simulink model "carry_ripple_adder"  (R2022b)
settings: Solver=FixedStepDiscrete  StartTime=0.0  StopTime=10  RelTol=1e-3
PreLoadFcn:
  | addpath('C:\Course_Material\UofT\ECE1718\assignment2\matlab_tests\hdlimport\carry_ripple_adder');
libraries: simulink x188, hdlsllib x65
(part 1 of 2)
CloseFcn:
  | addpath('C:\Course_Material\UofT\ECE1718\assignment2\matlab_tests\hdlimport\carry_ripple_adder');
  | rmpath('C:\Course_Material\UofT\ECE1718\assignment2\matlab_tests\hdlimport\carry_ripple_adder');
settings Model: DataTypeOverride=Off  Creator=13698  LastModifiedBy=13698
settings OptimizationCC: BlockReduction=off  ConditionallyExecuteInputs=off  DefaultParameterBehavior=Inlined  InheritOutputTypeSmallerThanSingle=on
settings DebuggingCC: AlgebraicLoopMsg=error  InheritedTsInSrcMsg=none  SingleTaskRateTransMsg=error
settings HardwareCC: ProdBitPerPointer=32  ProdBitPerSizeT=32  ProdBitPerPtrDiffT=32  ProdLargestAtomicFloat=None  ProdIntDivRoundTo=Undefined  ProdEndianess=Unspecified  ProdWordSize=32  ProdHWDeviceType=ASIC/FPGA->ASIC/FPGA  TargetBitPerPointer=64  TargetBitPerSizeT=64  TargetBitPerPtrDiffT=64  TargetLongLongMode=on  TargetIntDivRoundTo=Zero  TargetEndianess=LittleEndian  TargetWordSize=64  TargetHWDeviceType=Custom Processor->MATLAB Host Computer  ProdEqTarget=off

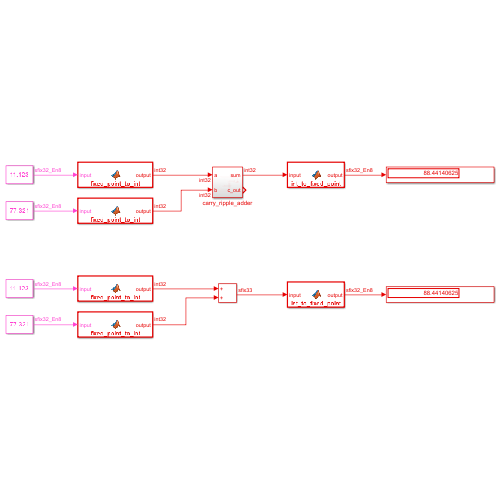
[thumbnail: Simulink's stored preview of the top-level diagram]
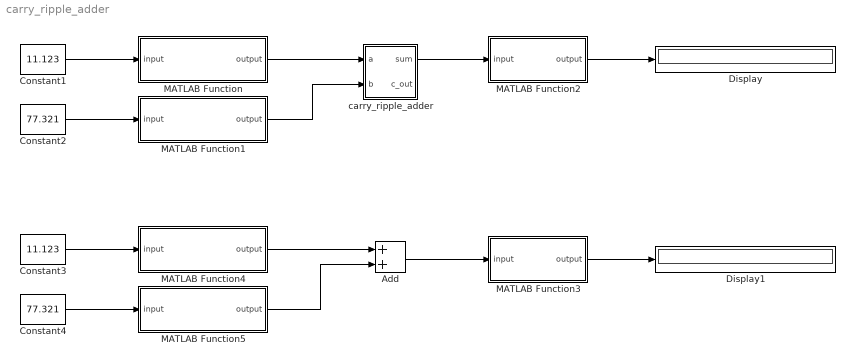
== system carry_ripple_adder ==
  Add : Sum
  Constant1 : Constant  Value=11.123  OutDataTypeStr=fixdt(1,32,8)
  Constant2 : Constant  Value=77.321  OutDataTypeStr=fixdt(1,32,8)
  Constant3 : Constant  Value=11.123  OutDataTypeStr=fixdt(1,32,8)
  Constant4 : Constant  Value=77.321  OutDataTypeStr=fixdt(1,32,8)
  Display : Display
  Display1 : Display
  MATLAB Function : MATLAB Function  TreatAsAtomicUnit=on
  MATLAB Function1 : MATLAB Function  TreatAsAtomicUnit=on
  MATLAB Function2 : MATLAB Function  TreatAsAtomicUnit=on
  MATLAB Function3 : MATLAB Function  TreatAsAtomicUnit=on
  MATLAB Function4 : MATLAB Function  TreatAsAtomicUnit=on
  MATLAB Function5 : MATLAB Function  TreatAsAtomicUnit=on
  carry_ripple_adder : Subsystem
  wires:
  MATLAB Function/1(output) -> carry_ripple_adder/1(a)
  MATLAB Function1/1(output) -> carry_ripple_adder/2(b)
  carry_ripple_adder/1(sum) -> MATLAB Function2/1(input)
  Constant1/1 -> MATLAB Function/1(input)
  MATLAB Function2/1(output) -> Display/1
  Add/1 -> MATLAB Function3/1(input)
  MATLAB Function3/1(output) -> Display1/1
  Constant3/1 -> MATLAB Function4/1(input)
  MATLAB Function4/1(output) -> Add/1
  MATLAB Function5/1(output) -> Add/2
  Constant2/1 -> MATLAB Function1/1(input)
  Constant4/1 -> MATLAB Function5/1(input)

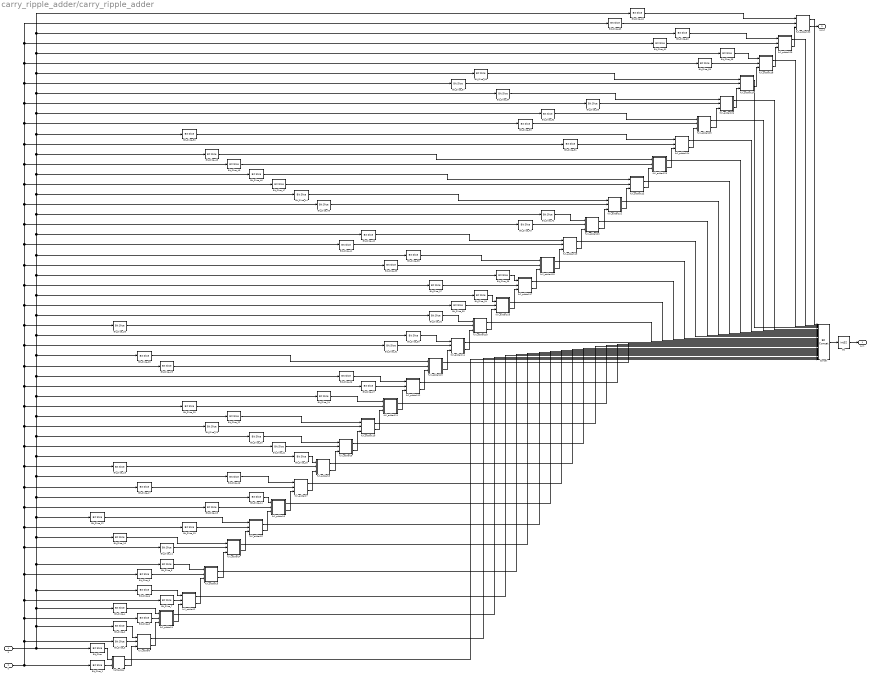
== system carry_ripple_adder/carry_ripple_adder ==
  a : Inport  OutDataTypeStr=int32  SampleTime=-1
  b : Inport  Port=2  OutDataTypeStr=int32  SampleTime=-1
  Bit_Slice : hdlsllib/Logic and Bit Operations/Bit Slice  lidx=double(0)  ridx=double(0)
  Bit_Slice_1 : hdlsllib/Logic and Bit Operations/Bit Slice  lidx=double(0)  ridx=double(0)
  Bit_Slice_10 : hdlsllib/Logic and Bit Operations/Bit Slice  lidx=double(5)  ridx=double(5)
  Bit_Slice_11 : hdlsllib/Logic and Bit Operations/Bit Slice  lidx=double(5)  ridx=double(5)
  Bit_Slice_12 : hdlsllib/Logic and Bit Operations/Bit Slice  lidx=double(6)  ridx=double(6)
  Bit_Slice_13 : hdlsllib/Logic and Bit Operations/Bit Slice  lidx=double(6)  ridx=double(6)
  Bit_Slice_14 : hdlsllib/Logic and Bit Operations/Bit Slice  lidx=double(7)  ridx=double(7)
  Bit_Slice_15 : hdlsllib/Logic and Bit Operations/Bit Slice  lidx=double(7)  ridx=double(7)
  Bit_Slice_16 : hdlsllib/Logic and Bit Operations/Bit Slice  lidx=double(8)  ridx=double(8)
  Bit_Slice_17 : hdlsllib/Logic and Bit Operations/Bit Slice  lidx=double(8)  ridx=double(8)
  Bit_Slice_18 : hdlsllib/Logic and Bit Operations/Bit Slice  lidx=double(9)  ridx=double(9)
  Bit_Slice_19 : hdlsllib/Logic and Bit Operations/Bit Slice  lidx=double(9)  ridx=double(9)
  Bit_Slice_2 : hdlsllib/Logic and Bit Operations/Bit Slice  lidx=double(1)  ridx=double(1)
  Bit_Slice_20 : hdlsllib/Logic and Bit Operations/Bit Slice  lidx=double(10)  ridx=double(10)
  Bit_Slice_21 : hdlsllib/Logic and Bit Operations/Bit Slice  lidx=double(10)  ridx=double(10)
  Bit_Slice_22 : hdlsllib/Logic and Bit Operations/Bit Slice  lidx=double(11)  ridx=double(11)
  Bit_Slice_23 : hdlsllib/Logic and Bit Operations/Bit Slice  lidx=double(11)  ridx=double(11)
  Bit_Slice_24 : hdlsllib/Logic and Bit Operations/Bit Slice  lidx=double(12)  ridx=double(12)
  Bit_Slice_25 : hdlsllib/Logic and Bit Operations/Bit Slice  lidx=double(12)  ridx=double(12)
  Bit_Slice_26 : hdlsllib/Logic and Bit Operations/Bit Slice  lidx=double(13)  ridx=double(13)
  Bit_Slice_27 : hdlsllib/Logic and Bit Operations/Bit Slice  lidx=double(13)  ridx=double(13)
  Bit_Slice_28 : hdlsllib/Logic and Bit Operations/Bit Slice  lidx=double(14)  ridx=double(14)
  Bit_Slice_29 : hdlsllib/Logic and Bit Operations/Bit Slice  lidx=double(14)  ridx=double(14)
  Bit_Slice_3 : hdlsllib/Logic and Bit Operations/Bit Slice  lidx=double(1)  ridx=double(1)
  Bit_Slice_30 : hdlsllib/Logic and Bit Operations/Bit Slice  lidx=double(15)  ridx=double(15)
  Bit_Slice_31 : hdlsllib/Logic and Bit Operations/Bit Slice  lidx=double(15)  ridx=double(15)
  Bit_Slice_32 : hdlsllib/Logic and Bit Operations/Bit Slice  lidx=double(16)  ridx=double(16)
  Bit_Slice_33 : hdlsllib/Logic and Bit Operations/Bit Slice  lidx=double(16)  ridx=double(16)
  Bit_Slice_34 : hdlsllib/Logic and Bit Operations/Bit Slice  lidx=double(17)  ridx=double(17)
  Bit_Slice_35 : hdlsllib/Logic and Bit Operations/Bit Slice  lidx=double(17)  ridx=double(17)
  Bit_Slice_36 : hdlsllib/Logic and Bit Operations/Bit Slice  lidx=double(18)  ridx=double(18)
  Bit_Slice_37 : hdlsllib/Logic and Bit Operations/Bit Slice  lidx=double(18)  ridx=double(18)
  Bit_Slice_38 : hdlsllib/Logic and Bit Operations/Bit Slice  lidx=double(19)  ridx=double(19)
  Bit_Slice_39 : hdlsllib/Logic and Bit Operations/Bit Slice  lidx=double(19)  ridx=double(19)
  Bit_Slice_4 : hdlsllib/Logic and Bit Operations/Bit Slice  lidx=double(2)  ridx=double(2)
  Bit_Slice_40 : hdlsllib/Logic and Bit Operations/Bit Slice  lidx=double(20)  ridx=double(20)
  Bit_Slice_41 : hdlsllib/Logic and Bit Operations/Bit Slice  lidx=double(20)  ridx=double(20)
  Bit_Slice_42 : hdlsllib/Logic and Bit Operations/Bit Slice  lidx=double(21)  ridx=double(21)
  Bit_Slice_43 : hdlsllib/Logic and Bit Operations/Bit Slice  lidx=double(21)  ridx=double(21)
  Bit_Slice_44 : hdlsllib/Logic and Bit Operations/Bit Slice  lidx=double(22)  ridx=double(22)
  Bit_Slice_45 : hdlsllib/Logic and Bit Operations/Bit Slice  lidx=double(22)  ridx=double(22)
  Bit_Slice_46 : hdlsllib/Logic and Bit Operations/Bit Slice  lidx=double(23)  ridx=double(23)
  Bit_Slice_47 : hdlsllib/Logic and Bit Operations/Bit Slice  lidx=double(23)  ridx=double(23)
  Bit_Slice_48 : hdlsllib/Logic and Bit Operations/Bit Slice  lidx=double(24)  ridx=double(24)
  Bit_Slice_49 : hdlsllib/Logic and Bit Operations/Bit Slice  lidx=double(24)  ridx=double(24)
  Bit_Slice_5 : hdlsllib/Logic and Bit Operations/Bit Slice  lidx=double(2)  ridx=double(2)
  Bit_Slice_50 : hdlsllib/Logic and Bit Operations/Bit Slice  lidx=double(25)  ridx=double(25)
  Bit_Slice_51 : hdlsllib/Logic and Bit Operations/Bit Slice  lidx=double(25)  ridx=double(25)
  Bit_Slice_52 : hdlsllib/Logic and Bit Operations/Bit Slice  lidx=double(26)  ridx=double(26)
  Bit_Slice_53 : hdlsllib/Logic and Bit Operations/Bit Slice  lidx=double(26)  ridx=double(26)
  Bit_Slice_54 : hdlsllib/Logic and Bit Operations/Bit Slice  lidx=double(27)  ridx=double(27)
  Bit_Slice_55 : hdlsllib/Logic and Bit Operations/Bit Slice  lidx=double(27)  ridx=double(27)
  Bit_Slice_56 : hdlsllib/Logic and Bit Operations/Bit Slice  lidx=double(28)  ridx=double(28)
  Bit_Slice_57 : hdlsllib/Logic and Bit Operations/Bit Slice  lidx=double(28)  ridx=double(28)
  Bit_Slice_58 : hdlsllib/Logic and Bit Operations/Bit Slice  lidx=double(29)  ridx=double(29)
  Bit_Slice_59 : hdlsllib/Logic and Bit Operations/Bit Slice  lidx=double(29)  ridx=double(29)
  Bit_Slice_6 : hdlsllib/Logic and Bit Operations/Bit Slice  lidx=double(3)  ridx=double(3)
  Bit_Slice_60 : hdlsllib/Logic and Bit Operations/Bit Slice  lidx=double(30)  ridx=double(30)
  Bit_Slice_61 : hdlsllib/Logic and Bit Operations/Bit Slice  lidx=double(30)  ridx=double(30)
  Bit_Slice_62 : hdlsllib/Logic and Bit Operations/Bit Slice  lidx=double(31)  ridx=double(31)
  Bit_Slice_63 : hdlsllib/Logic and Bit Operations/Bit Slice  lidx=double(31)  ridx=double(31)
  Bit_Slice_7 : hdlsllib/Logic and Bit Operations/Bit Slice  lidx=double(3)  ridx=double(3)
  Bit_Slice_8 : hdlsllib/Logic and Bit Operations/Bit Slice  lidx=double(4)  ridx=double(4)
  Bit_Slice_9 : hdlsllib/Logic and Bit Operations/Bit Slice  lidx=double(4)  ridx=double(4)
  Concat : hdlsllib/Logic and Bit Operations/Bit Concat  numInputs=32
  dtc : DataTypeConversion  OutDataTypeStr=int32  ConvertRealWorld=Stored Integer (SI)  SampleTime=-1  SaturateOnIntegerOverflow=off  RndMeth=Floor
  full_adder0 : Subsystem
  full_adder11 : Subsystem
  full_adder110 : Subsystem
  full_adder111 : Subsystem
  full_adder112 : Subsystem
  full_adder113 : Subsystem
  full_adder114 : Subsystem
  full_adder115 : Subsystem
  full_adder116 : Subsystem
  full_adder117 : Subsystem
  full_adder118 : Subsystem
  full_adder119 : Subsystem
  full_adder12 : Subsystem
  full_adder120 : Subsystem
  full_adder121 : Subsystem
  full_adder122 : Subsystem
  full_adder123 : Subsystem
  full_adder124 : Subsystem
  full_adder125 : Subsystem
  full_adder126 : Subsystem
  full_adder127 : Subsystem
  full_adder128 : Subsystem
  full_adder129 : Subsystem
  full_adder13 : Subsystem
  full_adder130 : Subsystem
  full_adder14 : Subsystem
  full_adder15 : Subsystem
  full_adder16 : Subsystem
  full_adder17 : Subsystem
  full_adder18 : Subsystem
  full_adder19 : Subsystem
  half_adder : Subsystem
  sum : Outport  OutDataTypeStr=int32  SampleTime=-1
  c_out : Outport  Port=2  OutDataTypeStr=fixdt(0, 1, 0)  SampleTime=-1
  wires:
  Bit_Slice/1 -> half_adder/1(a)
  full_adder122/2(c_out) -> full_adder123/3(c_in)
  full_adder130/2(c_out) -> c_out/1
  full_adder118/1(sum) -> Concat/13
  full_adder130/1(sum) -> Concat/1
  Bit_Slice_7/1 -> full_adder12/2(b)
  full_adder129/2(c_out) -> full_adder130/3(c_in)
  full_adder0/1(sum) -> Concat/31
  full_adder124/2(c_out) -> full_adder125/3(c_in)
  Concat/1 -> dtc/1
  Bit_Slice_20/1 -> full_adder19/1(a)
  full_adder14/2(c_out) -> full_adder15/3(c_in)
  full_adder117/2(c_out) -> full_adder118/3(c_in)
  full_adder121/2(c_out) -> full_adder122/3(c_in)
  full_adder120/1(sum) -> Concat/11
  full_adder116/1(sum) -> Concat/15
  Bit_Slice_51/1 -> full_adder124/2(b)
  full_adder128/2(c_out) -> full_adder129/3(c_in)
  Bit_Slice_36/1 -> full_adder117/1(a)
  Bit_Slice_28/1 -> full_adder113/1(a)
  Bit_Slice_16/1 -> full_adder17/1(a)
  full_adder120/2(c_out) -> full_adder121/3(c_in)
  full_adder125/2(c_out) -> full_adder126/3(c_in)
  full_adder118/2(c_out) -> full_adder119/3(c_in)
  full_adder12/1(sum) -> Concat/29
  Bit_Slice_18/1 -> full_adder18/1(a)
  full_adder127/2(c_out) -> full_adder128/3(c_in)
  full_adder19/2(c_out) -> full_adder110/3(c_in)
  full_adder126/2(c_out) -> full_adder127/3(c_in)
  full_adder12/2(c_out) -> full_adder13/3(c_in)
  Bit_Slice_14/1 -> full_adder16/1(a)
  full_adder110/2(c_out) -> full_adder111/3(c_in)
  b/1 -> Bit_Slice_63/1, Bit_Slice_61/1, Bit_Slice_59/1, Bit_Slice_57/1, Bit_Slice_55/1, Bit_Slice_53/1, Bit_Slice_51/1, Bit_Slice_49/1, Bit_Slice_47/1, Bit_Slice_45/1, Bit_Slice_43/1, Bit_Slice_41/1, Bit_Slice_39/1, Bit_Slice_37/1, Bit_Slice_35/1, Bit_Slice_33/1, Bit_Slice_31/1, Bit_Slice_29/1, Bit_Slice_27/1, Bit_Slice_25/1, Bit_Slice_23/1, Bit_Slice_21/1, Bit_Slice_19/1, Bit_Slice_17/1, Bit_Slice_15/1, Bit_Slice_13/1, Bit_Slice_11/1, Bit_Slice_9/1, Bit_Slice_7/1, Bit_Slice_5/1, Bit_Slice_3/1, Bit_Slice_1/1
  full_adder119/1(sum) -> Concat/12
  Bit_Slice_34/1 -> full_adder116/1(a)
  full_adder123/2(c_out) -> full_adder124/3(c_in)
  full_adder119/2(c_out) -> full_adder120/3(c_in)
  full_adder0/2(c_out) -> full_adder11/3(c_in)
  a/1 -> Bit_Slice_62/1, Bit_Slice_60/1, Bit_Slice_58/1, Bit_Slice_56/1, Bit_Slice_54/1, Bit_Slice_52/1, Bit_Slice_50/1, Bit_Slice_48/1, Bit_Slice_46/1, Bit_Slice_44/1, Bit_Slice_42/1, Bit_Slice_40/1, Bit_Slice_38/1, Bit_Slice_36/1, Bit_Slice_34/1, Bit_Slice_32/1, Bit_Slice_30/1, Bit_Slice_28/1, Bit_Slice_26/1, Bit_Slice_24/1, Bit_Slice_22/1, Bit_Slice_20/1, Bit_Slice_18/1, Bit_Slice_16/1, Bit_Slice_14/1, Bit_Slice_12/1, Bit_Slice_10/1, Bit_Slice_8/1, Bit_Slice_6/1, Bit_Slice_4/1, Bit_Slice_2/1, Bit_Slice/1
  full_adder116/2(c_out) -> full_adder117/3(c_in)
  Bit_Slice_46/1 -> full_adder122/1(a)
  Bit_Slice_2/1 -> full_adder0/1(a)
  full_adder115/2(c_out) -> full_adder116/3(c_in)
  Bit_Slice_33/1 -> full_adder115/2(b)
  full_adder112/2(c_out) -> full_adder113/3(c_in)
  Bit_Slice_13/1 -> full_adder15/2(b)
  full_adder114/2(c_out) -> full_adder115/3(c_in)
  full_adder113/2(c_out) -> full_adder114/3(c_in)
  full_adder111/2(c_out) -> full_adder112/3(c_in)
  full_adder18/2(c_out) -> full_adder19/3(c_in)
  full_adder123/1(sum) -> Concat/8
  full_adder17/2(c_out) -> full_adder18/3(c_in)
  full_adder13/2(c_out) -> full_adder14/3(c_in)
  Bit_Slice_9/1 -> full_adder13/2(b)
  full_adder16/2(c_out) -> full_adder17/3(c_in)
  full_adder15/2(c_out) -> full_adder16/3(c_in)
  Bit_Slice_3/1 -> full_adder0/2(b)
  full_adder11/2(c_out) -> full_adder12/3(c_in)
  Bit_Slice_5/1 -> full_adder11/2(b)
  Bit_Slice_1/1 -> half_adder/2(b)
  full_adder129/1(sum) -> Concat/2
  half_adder/2(c_out) -> full_adder0/3(c_in)
  full_adder17/1(sum) -> Concat/24
  dtc/1 -> sum/1
  full_adder113/1(sum) -> Concat/18
  Bit_Slice_31/1 -> full_adder114/2(b)
  full_adder124/1(sum) -> Concat/7
  Bit_Slice_10/1 -> full_adder14/1(a)
  Bit_Slice_12/1 -> full_adder15/1(a)
  Bit_Slice_17/1 -> full_adder17/2(b)
  Bit_Slice_19/1 -> full_adder18/2(b)
  Bit_Slice_4/1 -> full_adder11/1(a)
  half_adder/1(sum) -> Concat/32
  Bit_Slice_6/1 -> full_adder12/1(a)
  Bit_Slice_11/1 -> full_adder14/2(b)
  Bit_Slice_29/1 -> full_adder113/2(b)
  Bit_Slice_8/1 -> full_adder13/1(a)
  full_adder125/1(sum) -> Concat/6
  full_adder111/1(sum) -> Concat/20
  full_adder11/1(sum) -> Concat/30
  Bit_Slice_25/1 -> full_adder111/2(b)
  Bit_Slice_50/1 -> full_adder124/1(a)
  Bit_Slice_15/1 -> full_adder16/2(b)
  Bit_Slice_23/1 -> full_adder110/2(b)
  full_adder114/1(sum) -> Concat/17
  Bit_Slice_48/1 -> full_adder123/1(a)
  full_adder13/1(sum) -> Concat/28
  Bit_Slice_22/1 -> full_adder110/1(a)
  Bit_Slice_49/1 -> full_adder123/2(b)
  full_adder14/1(sum) -> Concat/27
  full_adder15/1(sum) -> Concat/26
  Bit_Slice_21/1 -> full_adder19/2(b)
  Bit_Slice_47/1 -> full_adder122/2(b)
  full_adder16/1(sum) -> Concat/25
  Bit_Slice_44/1 -> full_adder121/1(a)
  Bit_Slice_24/1 -> full_adder111/1(a)
  Bit_Slice_45/1 -> full_adder121/2(b)
  full_adder18/1(sum) -> Concat/23
  Bit_Slice_26/1 -> full_adder112/1(a)
  Bit_Slice_41/1 -> full_adder119/2(b)
  full_adder110/1(sum) -> Concat/21
  full_adder19/1(sum) -> Concat/22
  Bit_Slice_27/1 -> full_adder112/2(b)
  Bit_Slice_40/1 -> full_adder119/1(a)
  Bit_Slice_61/1 -> full_adder129/2(b)
  Bit_Slice_39/1 -> full_adder118/2(b)
  Bit_Slice_30/1 -> full_adder114/1(a)
  Bit_Slice_38/1 -> full_adder118/1(a)
  full_adder112/1(sum) -> Concat/19
  Bit_Slice_63/1 -> full_adder130/2(b)
  Bit_Slice_32/1 -> full_adder115/1(a)
  Bit_Slice_37/1 -> full_adder117/2(b)
  Bit_Slice_35/1 -> full_adder116/2(b)
  Bit_Slice_57/1 -> full_adder127/2(b)
  Bit_Slice_56/1 -> full_adder127/1(a)
  Bit_Slice_58/1 -> full_adder128/1(a)
  full_adder115/1(sum) -> Concat/16
  Bit_Slice_54/1 -> full_adder126/1(a)
  Bit_Slice_43/1 -> full_adder120/2(b)
  Bit_Slice_53/1 -> full_adder125/2(b)
  full_adder117/1(sum) -> Concat/14
  Bit_Slice_42/1 -> full_adder120/1(a)
  Bit_Slice_52/1 -> full_adder125/1(a)
  Bit_Slice_60/1 -> full_adder129/1(a)
  Bit_Slice_55/1 -> full_adder126/2(b)
  full_adder121/1(sum) -> Concat/10
  Bit_Slice_62/1 -> full_adder130/1(a)
  full_adder122/1(sum) -> Concat/9
  Bit_Slice_59/1 -> full_adder128/2(b)
  full_adder126/1(sum) -> Concat/5
  full_adder127/1(sum) -> Concat/4
  full_adder128/1(sum) -> Concat/3

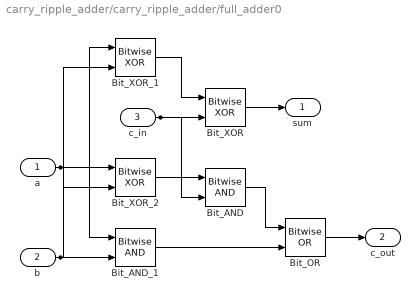
== system carry_ripple_adder/carry_ripple_adder/full_adder0 ==
  a : Inport  OutDataTypeStr=fixdt(0, 1, 0)  SampleTime=-1
  b : Inport  Port=2  OutDataTypeStr=fixdt(0, 1, 0)  SampleTime=-1
  c_in : Inport  Port=3  OutDataTypeStr=fixdt(0, 1, 0)  SampleTime=-1
  Bit_AND : simulink/Logic and Bit Operations/Bitwise Operator  logicop=AND  UseBitMask=off  NumInputPorts=2  BitMask=double(0)  BitMaskRealWorld=Real World Value
  Bit_AND_1 : simulink/Logic and Bit Operations/Bitwise Operator  logicop=AND  UseBitMask=off  NumInputPorts=2  BitMask=double(0)  BitMaskRealWorld=Real World Value
  Bit_OR : simulink/Logic and Bit Operations/Bitwise Operator  logicop=OR  UseBitMask=off  NumInputPorts=2  BitMask=double(0)  BitMaskRealWorld=Real World Value
  Bit_XOR : simulink/Logic and Bit Operations/Bitwise Operator  logicop=XOR  UseBitMask=off  NumInputPorts=2  BitMask=double(0)  BitMaskRealWorld=Real World Value
  Bit_XOR_1 : simulink/Logic and Bit Operations/Bitwise Operator  logicop=XOR  UseBitMask=off  NumInputPorts=2  BitMask=double(0)  BitMaskRealWorld=Real World Value
  Bit_XOR_2 : simulink/Logic and Bit Operations/Bitwise Operator  logicop=XOR  UseBitMask=off  NumInputPorts=2  BitMask=double(0)  BitMaskRealWorld=Real World Value
  sum : Outport  OutDataTypeStr=fixdt(0, 1, 0)  SampleTime=-1
  c_out : Outport  Port=2  OutDataTypeStr=fixdt(0, 1, 0)  SampleTime=-1
  wires:
  a/1 -> Bit_XOR_2/1, Bit_XOR_1/1, Bit_AND_1/1
  b/1 -> Bit_AND_1/2, Bit_XOR_2/2, Bit_XOR_1/2
  Bit_AND/1 -> Bit_OR/1
  Bit_XOR/1 -> sum/1
  Bit_AND_1/1 -> Bit_OR/2
  Bit_XOR_2/1 -> Bit_AND/1
  Bit_XOR_1/1 -> Bit_XOR/1
  c_in/1 -> Bit_AND/2, Bit_XOR/2
  Bit_OR/1 -> c_out/1

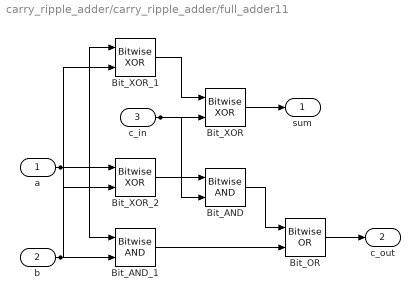
== system carry_ripple_adder/carry_ripple_adder/full_adder11 ==
  a : Inport  OutDataTypeStr=fixdt(0, 1, 0)  SampleTime=-1
  b : Inport  Port=2  OutDataTypeStr=fixdt(0, 1, 0)  SampleTime=-1
  c_in : Inport  Port=3  OutDataTypeStr=fixdt(0, 1, 0)  SampleTime=-1
  Bit_AND : simulink/Logic and Bit Operations/Bitwise Operator  logicop=AND  UseBitMask=off  NumInputPorts=2  BitMask=double(0)  BitMaskRealWorld=Real World Value
  Bit_AND_1 : simulink/Logic and Bit Operations/Bitwise Operator  logicop=AND  UseBitMask=off  NumInputPorts=2  BitMask=double(0)  BitMaskRealWorld=Real World Value
  Bit_OR : simulink/Logic and Bit Operations/Bitwise Operator  logicop=OR  UseBitMask=off  NumInputPorts=2  BitMask=double(0)  BitMaskRealWorld=Real World Value
  Bit_XOR : simulink/Logic and Bit Operations/Bitwise Operator  logicop=XOR  UseBitMask=off  NumInputPorts=2  BitMask=double(0)  BitMaskRealWorld=Real World Value
  Bit_XOR_1 : simulink/Logic and Bit Operations/Bitwise Operator  logicop=XOR  UseBitMask=off  NumInputPorts=2  BitMask=double(0)  BitMaskRealWorld=Real World Value
  Bit_XOR_2 : simulink/Logic and Bit Operations/Bitwise Operator  logicop=XOR  UseBitMask=off  NumInputPorts=2  BitMask=double(0)  BitMaskRealWorld=Real World Value
  sum : Outport  OutDataTypeStr=fixdt(0, 1, 0)  SampleTime=-1
  c_out : Outport  Port=2  OutDataTypeStr=fixdt(0, 1, 0)  SampleTime=-1
  wires:
  a/1 -> Bit_XOR_2/1, Bit_XOR_1/1, Bit_AND_1/1
  b/1 -> Bit_AND_1/2, Bit_XOR_2/2, Bit_XOR_1/2
  Bit_AND/1 -> Bit_OR/1
  Bit_XOR/1 -> sum/1
  Bit_AND_1/1 -> Bit_OR/2
  Bit_XOR_2/1 -> Bit_AND/1
  Bit_XOR_1/1 -> Bit_XOR/1
  c_in/1 -> Bit_AND/2, Bit_XOR/2
  Bit_OR/1 -> c_out/1

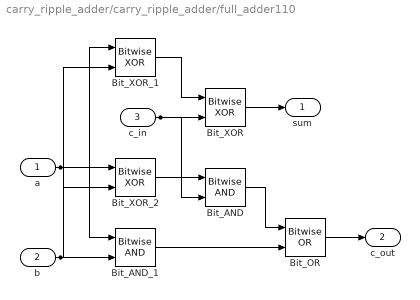
== system carry_ripple_adder/carry_ripple_adder/full_adder110 ==
  a : Inport  OutDataTypeStr=fixdt(0, 1, 0)  SampleTime=-1
  b : Inport  Port=2  OutDataTypeStr=fixdt(0, 1, 0)  SampleTime=-1
  c_in : Inport  Port=3  OutDataTypeStr=fixdt(0, 1, 0)  SampleTime=-1
  Bit_AND : simulink/Logic and Bit Operations/Bitwise Operator  logicop=AND  UseBitMask=off  NumInputPorts=2  BitMask=double(0)  BitMaskRealWorld=Real World Value
  Bit_AND_1 : simulink/Logic and Bit Operations/Bitwise Operator  logicop=AND  UseBitMask=off  NumInputPorts=2  BitMask=double(0)  BitMaskRealWorld=Real World Value
  Bit_OR : simulink/Logic and Bit Operations/Bitwise Operator  logicop=OR  UseBitMask=off  NumInputPorts=2  BitMask=double(0)  BitMaskRealWorld=Real World Value
  Bit_XOR : simulink/Logic and Bit Operations/Bitwise Operator  logicop=XOR  UseBitMask=off  NumInputPorts=2  BitMask=double(0)  BitMaskRealWorld=Real World Value
  Bit_XOR_1 : simulink/Logic and Bit Operations/Bitwise Operator  logicop=XOR  UseBitMask=off  NumInputPorts=2  BitMask=double(0)  BitMaskRealWorld=Real World Value
  Bit_XOR_2 : simulink/Logic and Bit Operations/Bitwise Operator  logicop=XOR  UseBitMask=off  NumInputPorts=2  BitMask=double(0)  BitMaskRealWorld=Real World Value
  sum : Outport  OutDataTypeStr=fixdt(0, 1, 0)  SampleTime=-1
  c_out : Outport  Port=2  OutDataTypeStr=fixdt(0, 1, 0)  SampleTime=-1
  wires:
  Bit_AND/1 -> Bit_OR/1
  Bit_XOR/1 -> sum/1
  Bit_AND_1/1 -> Bit_OR/2
  a/1 -> Bit_AND_1/1, Bit_XOR_2/1, Bit_XOR_1/1
  Bit_XOR_2/1 -> Bit_AND/1
  Bit_XOR_1/1 -> Bit_XOR/1
  b/1 -> Bit_AND_1/2, Bit_XOR_2/2, Bit_XOR_1/2
  c_in/1 -> Bit_AND/2, Bit_XOR/2
  Bit_OR/1 -> c_out/1

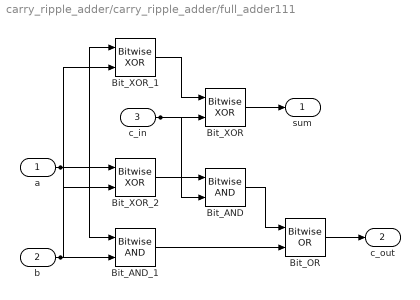
== system carry_ripple_adder/carry_ripple_adder/full_adder111 ==
  a : Inport  OutDataTypeStr=fixdt(0, 1, 0)  SampleTime=-1
  b : Inport  Port=2  OutDataTypeStr=fixdt(0, 1, 0)  SampleTime=-1
  c_in : Inport  Port=3  OutDataTypeStr=fixdt(0, 1, 0)  SampleTime=-1
  Bit_AND : simulink/Logic and Bit Operations/Bitwise Operator  logicop=AND  UseBitMask=off  NumInputPorts=2  BitMask=double(0)  BitMaskRealWorld=Real World Value
  Bit_AND_1 : simulink/Logic and Bit Operations/Bitwise Operator  logicop=AND  UseBitMask=off  NumInputPorts=2  BitMask=double(0)  BitMaskRealWorld=Real World Value
  Bit_OR : simulink/Logic and Bit Operations/Bitwise Operator  logicop=OR  UseBitMask=off  NumInputPorts=2  BitMask=double(0)  BitMaskRealWorld=Real World Value
  Bit_XOR : simulink/Logic and Bit Operations/Bitwise Operator  logicop=XOR  UseBitMask=off  NumInputPorts=2  BitMask=double(0)  BitMaskRealWorld=Real World Value
  Bit_XOR_1 : simulink/Logic and Bit Operations/Bitwise Operator  logicop=XOR  UseBitMask=off  NumInputPorts=2  BitMask=double(0)  BitMaskRealWorld=Real World Value
  Bit_XOR_2 : simulink/Logic and Bit Operations/Bitwise Operator  logicop=XOR  UseBitMask=off  NumInputPorts=2  BitMask=double(0)  BitMaskRealWorld=Real World Value
  sum : Outport  OutDataTypeStr=fixdt(0, 1, 0)  SampleTime=-1
  c_out : Outport  Port=2  OutDataTypeStr=fixdt(0, 1, 0)  SampleTime=-1
  wires:
  Bit_XOR/1 -> sum/1
  a/1 -> Bit_AND_1/1, Bit_XOR_2/1, Bit_XOR_1/1
  b/1 -> Bit_XOR_2/2, Bit_AND_1/2, Bit_XOR_1/2
  Bit_AND/1 -> Bit_OR/1
  Bit_AND_1/1 -> Bit_OR/2
  Bit_XOR_2/1 -> Bit_AND/1
  Bit_XOR_1/1 -> Bit_XOR/1
  c_in/1 -> Bit_AND/2, Bit_XOR/2
  Bit_OR/1 -> c_out/1

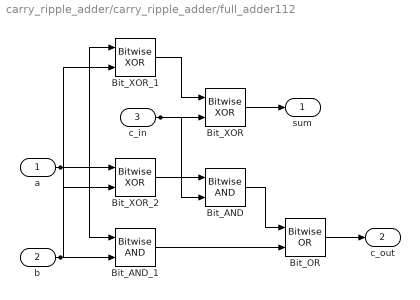
== system carry_ripple_adder/carry_ripple_adder/full_adder112 ==
  a : Inport  OutDataTypeStr=fixdt(0, 1, 0)  SampleTime=-1
  b : Inport  Port=2  OutDataTypeStr=fixdt(0, 1, 0)  SampleTime=-1
  c_in : Inport  Port=3  OutDataTypeStr=fixdt(0, 1, 0)  SampleTime=-1
  Bit_AND : simulink/Logic and Bit Operations/Bitwise Operator  logicop=AND  UseBitMask=off  NumInputPorts=2  BitMask=double(0)  BitMaskRealWorld=Real World Value
  Bit_AND_1 : simulink/Logic and Bit Operations/Bitwise Operator  logicop=AND  UseBitMask=off  NumInputPorts=2  BitMask=double(0)  BitMaskRealWorld=Real World Value
  Bit_OR : simulink/Logic and Bit Operations/Bitwise Operator  logicop=OR  UseBitMask=off  NumInputPorts=2  BitMask=double(0)  BitMaskRealWorld=Real World Value
  Bit_XOR : simulink/Logic and Bit Operations/Bitwise Operator  logicop=XOR  UseBitMask=off  NumInputPorts=2  BitMask=double(0)  BitMaskRealWorld=Real World Value
  Bit_XOR_1 : simulink/Logic and Bit Operations/Bitwise Operator  logicop=XOR  UseBitMask=off  NumInputPorts=2  BitMask=double(0)  BitMaskRealWorld=Real World Value
  Bit_XOR_2 : simulink/Logic and Bit Operations/Bitwise Operator  logicop=XOR  UseBitMask=off  NumInputPorts=2  BitMask=double(0)  BitMaskRealWorld=Real World Value
  sum : Outport  OutDataTypeStr=fixdt(0, 1, 0)  SampleTime=-1
  c_out : Outport  Port=2  OutDataTypeStr=fixdt(0, 1, 0)  SampleTime=-1
  wires:
  Bit_AND/1 -> Bit_OR/1
  Bit_XOR/1 -> sum/1
  Bit_AND_1/1 -> Bit_OR/2
  a/1 -> Bit_AND_1/1, Bit_XOR_2/1, Bit_XOR_1/1
  Bit_XOR_2/1 -> Bit_AND/1
  Bit_XOR_1/1 -> Bit_XOR/1
  b/1 -> Bit_AND_1/2, Bit_XOR_1/2, Bit_XOR_2/2
  c_in/1 -> Bit_AND/2, Bit_XOR/2
  Bit_OR/1 -> c_out/1

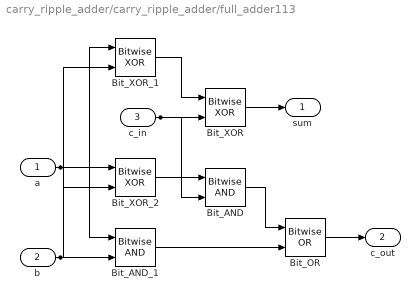
== system carry_ripple_adder/carry_ripple_adder/full_adder113 ==
  a : Inport  OutDataTypeStr=fixdt(0, 1, 0)  SampleTime=-1
  b : Inport  Port=2  OutDataTypeStr=fixdt(0, 1, 0)  SampleTime=-1
  c_in : Inport  Port=3  OutDataTypeStr=fixdt(0, 1, 0)  SampleTime=-1
  Bit_AND : simulink/Logic and Bit Operations/Bitwise Operator  logicop=AND  UseBitMask=off  NumInputPorts=2  BitMask=double(0)  BitMaskRealWorld=Real World Value
  Bit_AND_1 : simulink/Logic and Bit Operations/Bitwise Operator  logicop=AND  UseBitMask=off  NumInputPorts=2  BitMask=double(0)  BitMaskRealWorld=Real World Value
  Bit_OR : simulink/Logic and Bit Operations/Bitwise Operator  logicop=OR  UseBitMask=off  NumInputPorts=2  BitMask=double(0)  BitMaskRealWorld=Real World Value
  Bit_XOR : simulink/Logic and Bit Operations/Bitwise Operator  logicop=XOR  UseBitMask=off  NumInputPorts=2  BitMask=double(0)  BitMaskRealWorld=Real World Value
  Bit_XOR_1 : simulink/Logic and Bit Operations/Bitwise Operator  logicop=XOR  UseBitMask=off  NumInputPorts=2  BitMask=double(0)  BitMaskRealWorld=Real World Value
  Bit_XOR_2 : simulink/Logic and Bit Operations/Bitwise Operator  logicop=XOR  UseBitMask=off  NumInputPorts=2  BitMask=double(0)  BitMaskRealWorld=Real World Value
  sum : Outport  OutDataTypeStr=fixdt(0, 1, 0)  SampleTime=-1
  c_out : Outport  Port=2  OutDataTypeStr=fixdt(0, 1, 0)  SampleTime=-1
  wires:
  Bit_AND/1 -> Bit_OR/1
  Bit_XOR/1 -> sum/1
  Bit_XOR_1/1 -> Bit_XOR/1
  a/1 -> Bit_AND_1/1, Bit_XOR_2/1, Bit_XOR_1/1
  b/1 -> Bit_AND_1/2, Bit_XOR_2/2, Bit_XOR_1/2
  c_in/1 -> Bit_XOR/2, Bit_AND/2
  Bit_AND_1/1 -> Bit_OR/2
  Bit_XOR_2/1 -> Bit_AND/1
  Bit_OR/1 -> c_out/1

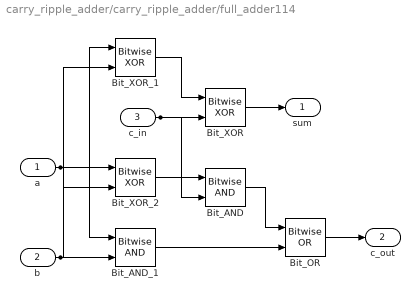
== system carry_ripple_adder/carry_ripple_adder/full_adder114 ==
  a : Inport  OutDataTypeStr=fixdt(0, 1, 0)  SampleTime=-1
  b : Inport  Port=2  OutDataTypeStr=fixdt(0, 1, 0)  SampleTime=-1
  c_in : Inport  Port=3  OutDataTypeStr=fixdt(0, 1, 0)  SampleTime=-1
  Bit_AND : simulink/Logic and Bit Operations/Bitwise Operator  logicop=AND  UseBitMask=off  NumInputPorts=2  BitMask=double(0)  BitMaskRealWorld=Real World Value
  Bit_AND_1 : simulink/Logic and Bit Operations/Bitwise Operator  logicop=AND  UseBitMask=off  NumInputPorts=2  BitMask=double(0)  BitMaskRealWorld=Real World Value
  Bit_OR : simulink/Logic and Bit Operations/Bitwise Operator  logicop=OR  UseBitMask=off  NumInputPorts=2  BitMask=double(0)  BitMaskRealWorld=Real World Value
  Bit_XOR : simulink/Logic and Bit Operations/Bitwise Operator  logicop=XOR  UseBitMask=off  NumInputPorts=2  BitMask=double(0)  BitMaskRealWorld=Real World Value
  Bit_XOR_1 : simulink/Logic and Bit Operations/Bitwise Operator  logicop=XOR  UseBitMask=off  NumInputPorts=2  BitMask=double(0)  BitMaskRealWorld=Real World Value
  Bit_XOR_2 : simulink/Logic and Bit Operations/Bitwise Operator  logicop=XOR  UseBitMask=off  NumInputPorts=2  BitMask=double(0)  BitMaskRealWorld=Real World Value
  sum : Outport  OutDataTypeStr=fixdt(0, 1, 0)  SampleTime=-1
  c_out : Outport  Port=2  OutDataTypeStr=fixdt(0, 1, 0)  SampleTime=-1
  wires:
  Bit_AND/1 -> Bit_OR/1
  Bit_XOR/1 -> sum/1
  Bit_AND_1/1 -> Bit_OR/2
  a/1 -> Bit_AND_1/1, Bit_XOR_1/1, Bit_XOR_2/1
  Bit_XOR_2/1 -> Bit_AND/1
  Bit_XOR_1/1 -> Bit_XOR/1
  b/1 -> Bit_AND_1/2, Bit_XOR_2/2, Bit_XOR_1/2
  c_in/1 -> Bit_AND/2, Bit_XOR/2
  Bit_OR/1 -> c_out/1

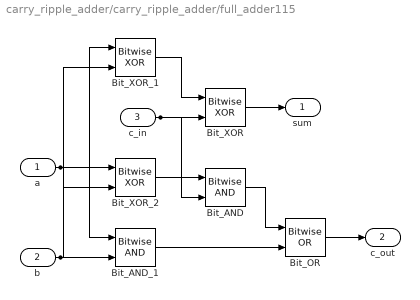
== system carry_ripple_adder/carry_ripple_adder/full_adder115 ==
  a : Inport  OutDataTypeStr=fixdt(0, 1, 0)  SampleTime=-1
  b : Inport  Port=2  OutDataTypeStr=fixdt(0, 1, 0)  SampleTime=-1
  c_in : Inport  Port=3  OutDataTypeStr=fixdt(0, 1, 0)  SampleTime=-1
  Bit_AND : simulink/Logic and Bit Operations/Bitwise Operator  logicop=AND  UseBitMask=off  NumInputPorts=2  BitMask=double(0)  BitMaskRealWorld=Real World Value
  Bit_AND_1 : simulink/Logic and Bit Operations/Bitwise Operator  logicop=AND  UseBitMask=off  NumInputPorts=2  BitMask=double(0)  BitMaskRealWorld=Real World Value
  Bit_OR : simulink/Logic and Bit Operations/Bitwise Operator  logicop=OR  UseBitMask=off  NumInputPorts=2  BitMask=double(0)  BitMaskRealWorld=Real World Value
  Bit_XOR : simulink/Logic and Bit Operations/Bitwise Operator  logicop=XOR  UseBitMask=off  NumInputPorts=2  BitMask=double(0)  BitMaskRealWorld=Real World Value
  Bit_XOR_1 : simulink/Logic and Bit Operations/Bitwise Operator  logicop=XOR  UseBitMask=off  NumInputPorts=2  BitMask=double(0)  BitMaskRealWorld=Real World Value
  Bit_XOR_2 : simulink/Logic and Bit Operations/Bitwise Operator  logicop=XOR  UseBitMask=off  NumInputPorts=2  BitMask=double(0)  BitMaskRealWorld=Real World Value
  sum : Outport  OutDataTypeStr=fixdt(0, 1, 0)  SampleTime=-1
  c_out : Outport  Port=2  OutDataTypeStr=fixdt(0, 1, 0)  SampleTime=-1
  wires:
  Bit_AND/1 -> Bit_OR/1
  Bit_XOR/1 -> sum/1
  Bit_AND_1/1 -> Bit_OR/2
  a/1 -> Bit_AND_1/1, Bit_XOR_2/1, Bit_XOR_1/1
  Bit_XOR_2/1 -> Bit_AND/1
  Bit_XOR_1/1 -> Bit_XOR/1
  b/1 -> Bit_XOR_2/2, Bit_XOR_1/2, Bit_AND_1/2
  c_in/1 -> Bit_AND/2, Bit_XOR/2
  Bit_OR/1 -> c_out/1

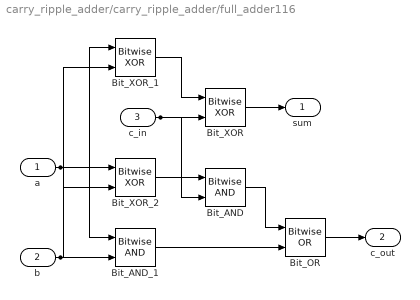
== system carry_ripple_adder/carry_ripple_adder/full_adder116 ==
  a : Inport  OutDataTypeStr=fixdt(0, 1, 0)  SampleTime=-1
  b : Inport  Port=2  OutDataTypeStr=fixdt(0, 1, 0)  SampleTime=-1
  c_in : Inport  Port=3  OutDataTypeStr=fixdt(0, 1, 0)  SampleTime=-1
  Bit_AND : simulink/Logic and Bit Operations/Bitwise Operator  logicop=AND  UseBitMask=off  NumInputPorts=2  BitMask=double(0)  BitMaskRealWorld=Real World Value
  Bit_AND_1 : simulink/Logic and Bit Operations/Bitwise Operator  logicop=AND  UseBitMask=off  NumInputPorts=2  BitMask=double(0)  BitMaskRealWorld=Real World Value
  Bit_OR : simulink/Logic and Bit Operations/Bitwise Operator  logicop=OR  UseBitMask=off  NumInputPorts=2  BitMask=double(0)  BitMaskRealWorld=Real World Value
  Bit_XOR : simulink/Logic and Bit Operations/Bitwise Operator  logicop=XOR  UseBitMask=off  NumInputPorts=2  BitMask=double(0)  BitMaskRealWorld=Real World Value
  Bit_XOR_1 : simulink/Logic and Bit Operations/Bitwise Operator  logicop=XOR  UseBitMask=off  NumInputPorts=2  BitMask=double(0)  BitMaskRealWorld=Real World Value
  Bit_XOR_2 : simulink/Logic and Bit Operations/Bitwise Operator  logicop=XOR  UseBitMask=off  NumInputPorts=2  BitMask=double(0)  BitMaskRealWorld=Real World Value
  sum : Outport  OutDataTypeStr=fixdt(0, 1, 0)  SampleTime=-1
  c_out : Outport  Port=2  OutDataTypeStr=fixdt(0, 1, 0)  SampleTime=-1
  wires:
  a/1 -> Bit_XOR_2/1, Bit_XOR_1/1, Bit_AND_1/1
  b/1 -> Bit_AND_1/2, Bit_XOR_2/2, Bit_XOR_1/2
  Bit_AND/1 -> Bit_OR/1
  Bit_XOR/1 -> sum/1
  Bit_AND_1/1 -> Bit_OR/2
  Bit_XOR_2/1 -> Bit_AND/1
  Bit_XOR_1/1 -> Bit_XOR/1
  c_in/1 -> Bit_AND/2, Bit_XOR/2
  Bit_OR/1 -> c_out/1

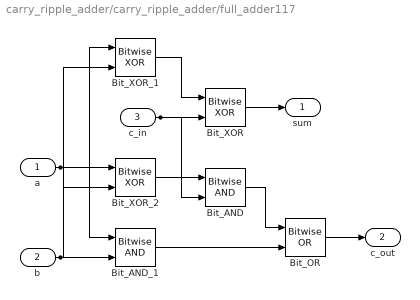
== system carry_ripple_adder/carry_ripple_adder/full_adder117 ==
  a : Inport  OutDataTypeStr=fixdt(0, 1, 0)  SampleTime=-1
  b : Inport  Port=2  OutDataTypeStr=fixdt(0, 1, 0)  SampleTime=-1
  c_in : Inport  Port=3  OutDataTypeStr=fixdt(0, 1, 0)  SampleTime=-1
  Bit_AND : simulink/Logic and Bit Operations/Bitwise Operator  logicop=AND  UseBitMask=off  NumInputPorts=2  BitMask=double(0)  BitMaskRealWorld=Real World Value
  Bit_AND_1 : simulink/Logic and Bit Operations/Bitwise Operator  logicop=AND  UseBitMask=off  NumInputPorts=2  BitMask=double(0)  BitMaskRealWorld=Real World Value
  Bit_OR : simulink/Logic and Bit Operations/Bitwise Operator  logicop=OR  UseBitMask=off  NumInputPorts=2  BitMask=double(0)  BitMaskRealWorld=Real World Value
  Bit_XOR : simulink/Logic and Bit Operations/Bitwise Operator  logicop=XOR  UseBitMask=off  NumInputPorts=2  BitMask=double(0)  BitMaskRealWorld=Real World Value
  Bit_XOR_1 : simulink/Logic and Bit Operations/Bitwise Operator  logicop=XOR  UseBitMask=off  NumInputPorts=2  BitMask=double(0)  BitMaskRealWorld=Real World Value
  Bit_XOR_2 : simulink/Logic and Bit Operations/Bitwise Operator  logicop=XOR  UseBitMask=off  NumInputPorts=2  BitMask=double(0)  BitMaskRealWorld=Real World Value
  sum : Outport  OutDataTypeStr=fixdt(0, 1, 0)  SampleTime=-1
  c_out : Outport  Port=2  OutDataTypeStr=fixdt(0, 1, 0)  SampleTime=-1
  wires:
  Bit_AND/1 -> Bit_OR/1
  Bit_XOR/1 -> sum/1
  Bit_AND_1/1 -> Bit_OR/2
  a/1 -> Bit_AND_1/1, Bit_XOR_2/1, Bit_XOR_1/1
  Bit_XOR_2/1 -> Bit_AND/1
  Bit_XOR_1/1 -> Bit_XOR/1
  b/1 -> Bit_AND_1/2, Bit_XOR_2/2, Bit_XOR_1/2
  c_in/1 -> Bit_AND/2, Bit_XOR/2
  Bit_OR/1 -> c_out/1

== system carry_ripple_adder/carry_ripple_adder/full_adder118 ==
  a : Inport  OutDataTypeStr=fixdt(0, 1, 0)  SampleTime=-1
  b : Inport  Port=2  OutDataTypeStr=fixdt(0, 1, 0)  SampleTime=-1
  c_in : Inport  Port=3  OutDataTypeStr=fixdt(0, 1, 0)  SampleTime=-1
  Bit_AND : simulink/Logic and Bit Operations/Bitwise Operator  logicop=AND  UseBitMask=off  NumInputPorts=2  BitMask=double(0)  BitMaskRealWorld=Real World Value
  Bit_AND_1 : simulink/Logic and Bit Operations/Bitwise Operator  logicop=AND  UseBitMask=off  NumInputPorts=2  BitMask=double(0)  BitMaskRealWorld=Real World Value
  Bit_OR : simulink/Logic and Bit Operations/Bitwise Operator  logicop=OR  UseBitMask=off  NumInputPorts=2  BitMask=double(0)  BitMaskRealWorld=Real World Value
  Bit_XOR : simulink/Logic and Bit Operations/Bitwise Operator  logicop=XOR  UseBitMask=off  NumInputPorts=2  BitMask=double(0)  BitMaskRealWorld=Real World Value
  Bit_XOR_1 : simulink/Logic and Bit Operations/Bitwise Operator  logicop=XOR  UseBitMask=off  NumInputPorts=2  BitMask=double(0)  BitMaskRealWorld=Real World Value
  Bit_XOR_2 : simulink/Logic and Bit Operations/Bitwise Operator  logicop=XOR  UseBitMask=off  NumInputPorts=2  BitMask=double(0)  BitMaskRealWorld=Real World Value
  sum : Outport  OutDataTypeStr=fixdt(0, 1, 0)  SampleTime=-1
  c_out : Outport  Port=2  OutDataTypeStr=fixdt(0, 1, 0)  SampleTime=-1
  wires:
  a/1 -> Bit_XOR_2/1, Bit_XOR_1/1, Bit_AND_1/1
  b/1 -> Bit_AND_1/2, Bit_XOR_2/2, Bit_XOR_1/2
  Bit_AND/1 -> Bit_OR/1
  Bit_XOR/1 -> sum/1
  Bit_AND_1/1 -> Bit_OR/2
  Bit_XOR_2/1 -> Bit_AND/1
  Bit_XOR_1/1 -> Bit_XOR/1
  c_in/1 -> Bit_AND/2, Bit_XOR/2
  Bit_OR/1 -> c_out/1

== system carry_ripple_adder/carry_ripple_adder/full_adder119 ==
  a : Inport  OutDataTypeStr=fixdt(0, 1, 0)  SampleTime=-1
  b : Inport  Port=2  OutDataTypeStr=fixdt(0, 1, 0)  SampleTime=-1
  c_in : Inport  Port=3  OutDataTypeStr=fixdt(0, 1, 0)  SampleTime=-1
  Bit_AND : simulink/Logic and Bit Operations/Bitwise Operator  logicop=AND  UseBitMask=off  NumInputPorts=2  BitMask=double(0)  BitMaskRealWorld=Real World Value
  Bit_AND_1 : simulink/Logic and Bit Operations/Bitwise Operator  logicop=AND  UseBitMask=off  NumInputPorts=2  BitMask=double(0)  BitMaskRealWorld=Real World Value
  Bit_OR : simulink/Logic and Bit Operations/Bitwise Operator  logicop=OR  UseBitMask=off  NumInputPorts=2  BitMask=double(0)  BitMaskRealWorld=Real World Value
  Bit_XOR : simulink/Logic and Bit Operations/Bitwise Operator  logicop=XOR  UseBitMask=off  NumInputPorts=2  BitMask=double(0)  BitMaskRealWorld=Real World Value
  Bit_XOR_1 : simulink/Logic and Bit Operations/Bitwise Operator  logicop=XOR  UseBitMask=off  NumInputPorts=2  BitMask=double(0)  BitMaskRealWorld=Real World Value
  Bit_XOR_2 : simulink/Logic and Bit Operations/Bitwise Operator  logicop=XOR  UseBitMask=off  NumInputPorts=2  BitMask=double(0)  BitMaskRealWorld=Real World Value
  sum : Outport  OutDataTypeStr=fixdt(0, 1, 0)  SampleTime=-1
  c_out : Outport  Port=2  OutDataTypeStr=fixdt(0, 1, 0)  SampleTime=-1
  wires:
  Bit_AND/1 -> Bit_OR/1
  Bit_XOR/1 -> sum/1
  Bit_AND_1/1 -> Bit_OR/2
  Bit_XOR_2/1 -> Bit_AND/1
  Bit_XOR_1/1 -> Bit_XOR/1
  a/1 -> Bit_AND_1/1, Bit_XOR_2/1, Bit_XOR_1/1
  b/1 -> Bit_AND_1/2, Bit_XOR_2/2, Bit_XOR_1/2
  c_in/1 -> Bit_XOR/2, Bit_AND/2
  Bit_OR/1 -> c_out/1

== system carry_ripple_adder/carry_ripple_adder/full_adder12 ==
  a : Inport  OutDataTypeStr=fixdt(0, 1, 0)  SampleTime=-1
  b : Inport  Port=2  OutDataTypeStr=fixdt(0, 1, 0)  SampleTime=-1
  c_in : Inport  Port=3  OutDataTypeStr=fixdt(0, 1, 0)  SampleTime=-1
  Bit_AND : simulink/Logic and Bit Operations/Bitwise Operator  logicop=AND  UseBitMask=off  NumInputPorts=2  BitMask=double(0)  BitMaskRealWorld=Real World Value
  Bit_AND_1 : simulink/Logic and Bit Operations/Bitwise Operator  logicop=AND  UseBitMask=off  NumInputPorts=2  BitMask=double(0)  BitMaskRealWorld=Real World Value
  Bit_OR : simulink/Logic and Bit Operations/Bitwise Operator  logicop=OR  UseBitMask=off  NumInputPorts=2  BitMask=double(0)  BitMaskRealWorld=Real World Value
  Bit_XOR : simulink/Logic and Bit Operations/Bitwise Operator  logicop=XOR  UseBitMask=off  NumInputPorts=2  BitMask=double(0)  BitMaskRealWorld=Real World Value
  Bit_XOR_1 : simulink/Logic and Bit Operations/Bitwise Operator  logicop=XOR  UseBitMask=off  NumInputPorts=2  BitMask=double(0)  BitMaskRealWorld=Real World Value
  Bit_XOR_2 : simulink/Logic and Bit Operations/Bitwise Operator  logicop=XOR  UseBitMask=off  NumInputPorts=2  BitMask=double(0)  BitMaskRealWorld=Real World Value
  sum : Outport  OutDataTypeStr=fixdt(0, 1, 0)  SampleTime=-1
  c_out : Outport  Port=2  OutDataTypeStr=fixdt(0, 1, 0)  SampleTime=-1
  wires:
  a/1 -> Bit_XOR_2/1, Bit_AND_1/1, Bit_XOR_1/1
  b/1 -> Bit_AND_1/2, Bit_XOR_2/2, Bit_XOR_1/2
  Bit_AND/1 -> Bit_OR/1
  Bit_XOR/1 -> sum/1
  Bit_AND_1/1 -> Bit_OR/2
  Bit_XOR_2/1 -> Bit_AND/1
  Bit_XOR_1/1 -> Bit_XOR/1
  c_in/1 -> Bit_XOR/2, Bit_AND/2
  Bit_OR/1 -> c_out/1

== system carry_ripple_adder/carry_ripple_adder/full_adder120 ==
  a : Inport  OutDataTypeStr=fixdt(0, 1, 0)  SampleTime=-1
  b : Inport  Port=2  OutDataTypeStr=fixdt(0, 1, 0)  SampleTime=-1
  c_in : Inport  Port=3  OutDataTypeStr=fixdt(0, 1, 0)  SampleTime=-1
  Bit_AND : simulink/Logic and Bit Operations/Bitwise Operator  logicop=AND  UseBitMask=off  NumInputPorts=2  BitMask=double(0)  BitMaskRealWorld=Real World Value
  Bit_AND_1 : simulink/Logic and Bit Operations/Bitwise Operator  logicop=AND  UseBitMask=off  NumInputPorts=2  BitMask=double(0)  BitMaskRealWorld=Real World Value
  Bit_OR : simulink/Logic and Bit Operations/Bitwise Operator  logicop=OR  UseBitMask=off  NumInputPorts=2  BitMask=double(0)  BitMaskRealWorld=Real World Value
  Bit_XOR : simulink/Logic and Bit Operations/Bitwise Operator  logicop=XOR  UseBitMask=off  NumInputPorts=2  BitMask=double(0)  BitMaskRealWorld=Real World Value
  Bit_XOR_1 : simulink/Logic and Bit Operations/Bitwise Operator  logicop=XOR  UseBitMask=off  NumInputPorts=2  BitMask=double(0)  BitMaskRealWorld=Real World Value
  Bit_XOR_2 : simulink/Logic and Bit Operations/Bitwise Operator  logicop=XOR  UseBitMask=off  NumInputPorts=2  BitMask=double(0)  BitMaskRealWorld=Real World Value
  sum : Outport  OutDataTypeStr=fixdt(0, 1, 0)  SampleTime=-1
  c_out : Outport  Port=2  OutDataTypeStr=fixdt(0, 1, 0)  SampleTime=-1
  wires:
  Bit_AND/1 -> Bit_OR/1
  Bit_XOR/1 -> sum/1
  Bit_AND_1/1 -> Bit_OR/2
  Bit_XOR_1/1 -> Bit_XOR/1
  a/1 -> Bit_AND_1/1, Bit_XOR_1/1, Bit_XOR_2/1
  Bit_XOR_2/1 -> Bit_AND/1
  b/1 -> Bit_XOR_2/2, Bit_AND_1/2, Bit_XOR_1/2
  c_in/1 -> Bit_AND/2, Bit_XOR/2
  Bit_OR/1 -> c_out/1

== system carry_ripple_adder/carry_ripple_adder/full_adder121 ==
  a : Inport  OutDataTypeStr=fixdt(0, 1, 0)  SampleTime=-1
  b : Inport  Port=2  OutDataTypeStr=fixdt(0, 1, 0)  SampleTime=-1
  c_in : Inport  Port=3  OutDataTypeStr=fixdt(0, 1, 0)  SampleTime=-1
  Bit_AND : simulink/Logic and Bit Operations/Bitwise Operator  logicop=AND  UseBitMask=off  NumInputPorts=2  BitMask=double(0)  BitMaskRealWorld=Real World Value
  Bit_AND_1 : simulink/Logic and Bit Operations/Bitwise Operator  logicop=AND  UseBitMask=off  NumInputPorts=2  BitMask=double(0)  BitMaskRealWorld=Real World Value
  Bit_OR : simulink/Logic and Bit Operations/Bitwise Operator  logicop=OR  UseBitMask=off  NumInputPorts=2  BitMask=double(0)  BitMaskRealWorld=Real World Value
  Bit_XOR : simulink/Logic and Bit Operations/Bitwise Operator  logicop=XOR  UseBitMask=off  NumInputPorts=2  BitMask=double(0)  BitMaskRealWorld=Real World Value
  Bit_XOR_1 : simulink/Logic and Bit Operations/Bitwise Operator  logicop=XOR  UseBitMask=off  NumInputPorts=2  BitMask=double(0)  BitMaskRealWorld=Real World Value
  Bit_XOR_2 : simulink/Logic and Bit Operations/Bitwise Operator  logicop=XOR  UseBitMask=off  NumInputPorts=2  BitMask=double(0)  BitMaskRealWorld=Real World Value
  sum : Outport  OutDataTypeStr=fixdt(0, 1, 0)  SampleTime=-1
  c_out : Outport  Port=2  OutDataTypeStr=fixdt(0, 1, 0)  SampleTime=-1
  wires:
  Bit_XOR/1 -> sum/1
  a/1 -> Bit_AND_1/1, Bit_XOR_2/1, Bit_XOR_1/1
  Bit_XOR_2/1 -> Bit_AND/1
  b/1 -> Bit_AND_1/2, Bit_XOR_2/2, Bit_XOR_1/2
  Bit_AND/1 -> Bit_OR/1
  Bit_AND_1/1 -> Bit_OR/2
  Bit_XOR_1/1 -> Bit_XOR/1
  c_in/1 -> Bit_AND/2, Bit_XOR/2
  Bit_OR/1 -> c_out/1

== system carry_ripple_adder/carry_ripple_adder/full_adder122 ==
  a : Inport  OutDataTypeStr=fixdt(0, 1, 0)  SampleTime=-1
  b : Inport  Port=2  OutDataTypeStr=fixdt(0, 1, 0)  SampleTime=-1
  c_in : Inport  Port=3  OutDataTypeStr=fixdt(0, 1, 0)  SampleTime=-1
  Bit_AND : simulink/Logic and Bit Operations/Bitwise Operator  logicop=AND  UseBitMask=off  NumInputPorts=2  BitMask=double(0)  BitMaskRealWorld=Real World Value
  Bit_AND_1 : simulink/Logic and Bit Operations/Bitwise Operator  logicop=AND  UseBitMask=off  NumInputPorts=2  BitMask=double(0)  BitMaskRealWorld=Real World Value
  Bit_OR : simulink/Logic and Bit Operations/Bitwise Operator  logicop=OR  UseBitMask=off  NumInputPorts=2  BitMask=double(0)  BitMaskRealWorld=Real World Value
  Bit_XOR : simulink/Logic and Bit Operations/Bitwise Operator  logicop=XOR  UseBitMask=off  NumInputPorts=2  BitMask=double(0)  BitMaskRealWorld=Real World Value
  Bit_XOR_1 : simulink/Logic and Bit Operations/Bitwise Operator  logicop=XOR  UseBitMask=off  NumInputPorts=2  BitMask=double(0)  BitMaskRealWorld=Real World Value
  Bit_XOR_2 : simulink/Logic and Bit Operations/Bitwise Operator  logicop=XOR  UseBitMask=off  NumInputPorts=2  BitMask=double(0)  BitMaskRealWorld=Real World Value
  sum : Outport  OutDataTypeStr=fixdt(0, 1, 0)  SampleTime=-1
  c_out : Outport  Port=2  OutDataTypeStr=fixdt(0, 1, 0)  SampleTime=-1
  wires:
  a/1 -> Bit_AND_1/1, Bit_XOR_2/1, Bit_XOR_1/1
  b/1 -> Bit_AND_1/2, Bit_XOR_1/2, Bit_XOR_2/2
  Bit_XOR_1/1 -> Bit_XOR/1
  Bit_AND_1/1 -> Bit_OR/2
  c_in/1 -> Bit_XOR/2, Bit_AND/2
  Bit_XOR_2/1 -> Bit_AND/1
  Bit_XOR/1 -> sum/1
  Bit_AND/1 -> Bit_OR/1
  Bit_OR/1 -> c_out/1

== system carry_ripple_adder/carry_ripple_adder/full_adder123 ==
  a : Inport  OutDataTypeStr=fixdt(0, 1, 0)  SampleTime=-1
  b : Inport  Port=2  OutDataTypeStr=fixdt(0, 1, 0)  SampleTime=-1
  c_in : Inport  Port=3  OutDataTypeStr=fixdt(0, 1, 0)  SampleTime=-1
  Bit_AND : simulink/Logic and Bit Operations/Bitwise Operator  logicop=AND  UseBitMask=off  NumInputPorts=2  BitMask=double(0)  BitMaskRealWorld=Real World Value
  Bit_AND_1 : simulink/Logic and Bit Operations/Bitwise Operator  logicop=AND  UseBitMask=off  NumInputPorts=2  BitMask=double(0)  BitMaskRealWorld=Real World Value
  Bit_OR : simulink/Logic and Bit Operations/Bitwise Operator  logicop=OR  UseBitMask=off  NumInputPorts=2  BitMask=double(0)  BitMaskRealWorld=Real World Value
  Bit_XOR : simulink/Logic and Bit Operations/Bitwise Operator  logicop=XOR  UseBitMask=off  NumInputPorts=2  BitMask=double(0)  BitMaskRealWorld=Real World Value
  Bit_XOR_1 : simulink/Logic and Bit Operations/Bitwise Operator  logicop=XOR  UseBitMask=off  NumInputPorts=2  BitMask=double(0)  BitMaskRealWorld=Real World Value
  Bit_XOR_2 : simulink/Logic and Bit Operations/Bitwise Operator  logicop=XOR  UseBitMask=off  NumInputPorts=2  BitMask=double(0)  BitMaskRealWorld=Real World Value
  sum : Outport  OutDataTypeStr=fixdt(0, 1, 0)  SampleTime=-1
  c_out : Outport  Port=2  OutDataTypeStr=fixdt(0, 1, 0)  SampleTime=-1
  wires:
  Bit_XOR/1 -> sum/1
  a/1 -> Bit_AND_1/1, Bit_XOR_2/1, Bit_XOR_1/1
  b/1 -> Bit_AND_1/2, Bit_XOR_2/2, Bit_XOR_1/2
  Bit_XOR_1/1 -> Bit_XOR/1
  Bit_AND/1 -> Bit_OR/1
  c_in/1 -> Bit_AND/2, Bit_XOR/2
  Bit_XOR_2/1 -> Bit_AND/1
  Bit_AND_1/1 -> Bit_OR/2
  Bit_OR/1 -> c_out/1

== system carry_ripple_adder/carry_ripple_adder/full_adder124 ==
  a : Inport  OutDataTypeStr=fixdt(0, 1, 0)  SampleTime=-1
  b : Inport  Port=2  OutDataTypeStr=fixdt(0, 1, 0)  SampleTime=-1
  c_in : Inport  Port=3  OutDataTypeStr=fixdt(0, 1, 0)  SampleTime=-1
  Bit_AND : simulink/Logic and Bit Operations/Bitwise Operator  logicop=AND  UseBitMask=off  NumInputPorts=2  BitMask=double(0)  BitMaskRealWorld=Real World Value
  Bit_AND_1 : simulink/Logic and Bit Operations/Bitwise Operator  logicop=AND  UseBitMask=off  NumInputPorts=2  BitMask=double(0)  BitMaskRealWorld=Real World Value
  Bit_OR : simulink/Logic and Bit Operations/Bitwise Operator  logicop=OR  UseBitMask=off  NumInputPorts=2  BitMask=double(0)  BitMaskRealWorld=Real World Value
  Bit_XOR : simulink/Logic and Bit Operations/Bitwise Operator  logicop=XOR  UseBitMask=off  NumInputPorts=2  BitMask=double(0)  BitMaskRealWorld=Real World Value
  Bit_XOR_1 : simulink/Logic and Bit Operations/Bitwise Operator  logicop=XOR  UseBitMask=off  NumInputPorts=2  BitMask=double(0)  BitMaskRealWorld=Real World Value
  Bit_XOR_2 : simulink/Logic and Bit Operations/Bitwise Operator  logicop=XOR  UseBitMask=off  NumInputPorts=2  BitMask=double(0)  BitMaskRealWorld=Real World Value
  sum : Outport  OutDataTypeStr=fixdt(0, 1, 0)  SampleTime=-1
  c_out : Outport  Port=2  OutDataTypeStr=fixdt(0, 1, 0)  SampleTime=-1
  wires:
  a/1 -> Bit_XOR_2/1, Bit_XOR_1/1, Bit_AND_1/1
  b/1 -> Bit_AND_1/2, Bit_XOR_2/2, Bit_XOR_1/2
  c_in/1 -> Bit_AND/2, Bit_XOR/2
  Bit_XOR_1/1 -> Bit_XOR/1
  Bit_XOR_2/1 -> Bit_AND/1
  Bit_AND_1/1 -> Bit_OR/2
  Bit_XOR/1 -> sum/1
  Bit_AND/1 -> Bit_OR/1
  Bit_OR/1 -> c_out/1

== system carry_ripple_adder/carry_ripple_adder/full_adder125 ==
  a : Inport  OutDataTypeStr=fixdt(0, 1, 0)  SampleTime=-1
  b : Inport  Port=2  OutDataTypeStr=fixdt(0, 1, 0)  SampleTime=-1
  c_in : Inport  Port=3  OutDataTypeStr=fixdt(0, 1, 0)  SampleTime=-1
  Bit_AND : simulink/Logic and Bit Operations/Bitwise Operator  logicop=AND  UseBitMask=off  NumInputPorts=2  BitMask=double(0)  BitMaskRealWorld=Real World Value
  Bit_AND_1 : simulink/Logic and Bit Operations/Bitwise Operator  logicop=AND  UseBitMask=off  NumInputPorts=2  BitMask=double(0)  BitMaskRealWorld=Real World Value
  Bit_OR : simulink/Logic and Bit Operations/Bitwise Operator  logicop=OR  UseBitMask=off  NumInputPorts=2  BitMask=double(0)  BitMaskRealWorld=Real World Value
  Bit_XOR : simulink/Logic and Bit Operations/Bitwise Operator  logicop=XOR  UseBitMask=off  NumInputPorts=2  BitMask=double(0)  BitMaskRealWorld=Real World Value
  Bit_XOR_1 : simulink/Logic and Bit Operations/Bitwise Operator  logicop=XOR  UseBitMask=off  NumInputPorts=2  BitMask=double(0)  BitMaskRealWorld=Real World Value
  Bit_XOR_2 : simulink/Logic and Bit Operations/Bitwise Operator  logicop=XOR  UseBitMask=off  NumInputPorts=2  BitMask=double(0)  BitMaskRealWorld=Real World Value
  sum : Outport  OutDataTypeStr=fixdt(0, 1, 0)  SampleTime=-1
  c_out : Outport  Port=2  OutDataTypeStr=fixdt(0, 1, 0)  SampleTime=-1
  wires:
  Bit_XOR/1 -> sum/1
  a/1 -> Bit_AND_1/1, Bit_XOR_2/1, Bit_XOR_1/1
  b/1 -> Bit_AND_1/2, Bit_XOR_2/2, Bit_XOR_1/2
  Bit_AND_1/1 -> Bit_OR/2
  Bit_XOR_1/1 -> Bit_XOR/1
  Bit_AND/1 -> Bit_OR/1
  c_in/1 -> Bit_AND/2, Bit_XOR/2
  Bit_XOR_2/1 -> Bit_AND/1
  Bit_OR/1 -> c_out/1

== system carry_ripple_adder/carry_ripple_adder/full_adder126 ==
  a : Inport  OutDataTypeStr=fixdt(0, 1, 0)  SampleTime=-1
  b : Inport  Port=2  OutDataTypeStr=fixdt(0, 1, 0)  SampleTime=-1
  c_in : Inport  Port=3  OutDataTypeStr=fixdt(0, 1, 0)  SampleTime=-1
  Bit_AND : simulink/Logic and Bit Operations/Bitwise Operator  logicop=AND  UseBitMask=off  NumInputPorts=2  BitMask=double(0)  BitMaskRealWorld=Real World Value
  Bit_AND_1 : simulink/Logic and Bit Operations/Bitwise Operator  logicop=AND  UseBitMask=off  NumInputPorts=2  BitMask=double(0)  BitMaskRealWorld=Real World Value
  Bit_OR : simulink/Logic and Bit Operations/Bitwise Operator  logicop=OR  UseBitMask=off  NumInputPorts=2  BitMask=double(0)  BitMaskRealWorld=Real World Value
  Bit_XOR : simulink/Logic and Bit Operations/Bitwise Operator  logicop=XOR  UseBitMask=off  NumInputPorts=2  BitMask=double(0)  BitMaskRealWorld=Real World Value
  Bit_XOR_1 : simulink/Logic and Bit Operations/Bitwise Operator  logicop=XOR  UseBitMask=off  NumInputPorts=2  BitMask=double(0)  BitMaskRealWorld=Real World Value
  Bit_XOR_2 : simulink/Logic and Bit Operations/Bitwise Operator  logicop=XOR  UseBitMask=off  NumInputPorts=2  BitMask=double(0)  BitMaskRealWorld=Real World Value
  sum : Outport  OutDataTypeStr=fixdt(0, 1, 0)  SampleTime=-1
  c_out : Outport  Port=2  OutDataTypeStr=fixdt(0, 1, 0)  SampleTime=-1
  wires:
  a/1 -> Bit_XOR_2/1, Bit_XOR_1/1, Bit_AND_1/1
  b/1 -> Bit_AND_1/2, Bit_XOR_1/2, Bit_XOR_2/2
  Bit_AND_1/1 -> Bit_OR/2
  Bit_XOR_1/1 -> Bit_XOR/1
  Bit_XOR/1 -> sum/1
  Bit_XOR_2/1 -> Bit_AND/1
  c_in/1 -> Bit_AND/2, Bit_XOR/2
  Bit_AND/1 -> Bit_OR/1
  Bit_OR/1 -> c_out/1
